simulink model "TwoScaleSimulation"  (R2021b)
settings: Solver=ode15s  StartTime=0.0  StopTime=1440*2  RelTol=1e-5
model workspace (MAT data in the model file):
  K_ACTH_StARp37 = 21.62
  k21 = 3080
  k_ACORT = 44.5
  k_StARp37 = 0.778
  ke = 0.099
  mu_StARp37 = 19.8
settings Model: Creator=Mahdi  LastModifiedBy=Mahdi
settings SolverCC: AlgebraicLoopSolver=TrustRegion
settings DebuggingCC: SFMachineParentedDataDiag=warning

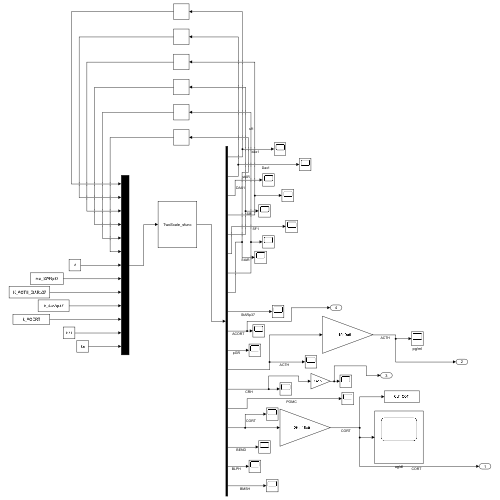
[thumbnail: Simulink's stored preview of the top-level diagram]
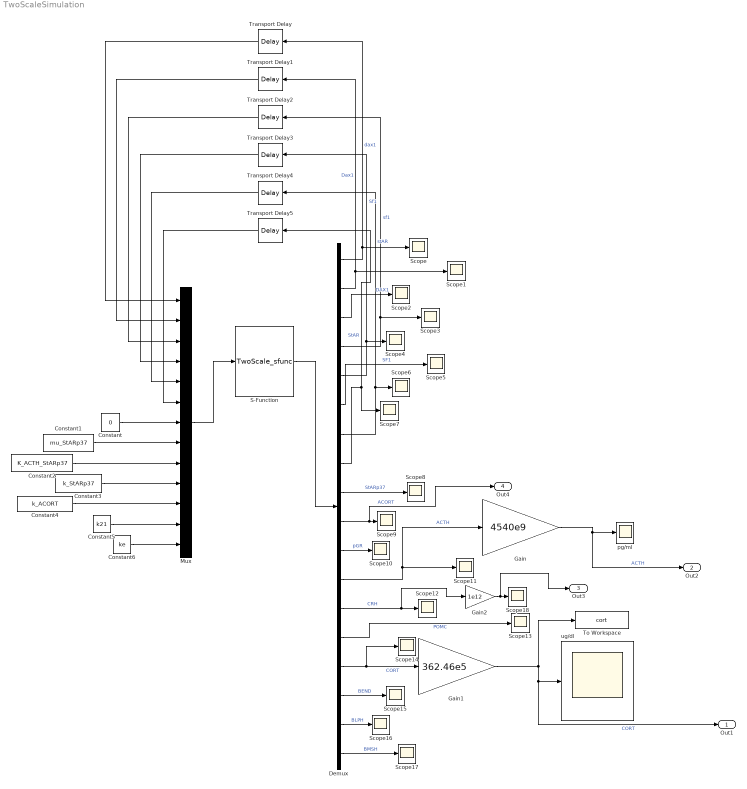
== system TwoScaleSimulation ==
  Constant : Constant  Value=0
  Constant1 : Constant  Value=mu_StARp37
  Constant2 : Constant  Value=K_ACTH_StARp37
  Constant3 : Constant  Value=k_StARp37
  Constant4 : Constant  Value=k_ACORT
  Constant5 : Constant  Value=k21
  Constant6 : Constant  Value=ke
  Demux : Demux  Outputs=18
  Gain : Gain  Gain=4540e9
  Gain1 : Gain  Gain=362.46e5
  Gain2 : Gain  Gain=1e12
  Mux : Mux  Inputs=13
  S-Function : S-Function  FunctionName=TwoScale_sfunc  SFunctionDeploymentMode=off  EnableBusSupport=off
  Scope{,1..18} (19 alike) : Scope
  To Workspace : ToWorkspace  VariableName=cort  SampleTime=10
  Transport Delay : TransportDelay  DelayTime=2.79
  Transport Delay1 : TransportDelay  DelayTime=1.4
  Transport Delay2 : TransportDelay  DelayTime=14.75
  Transport Delay3 : TransportDelay  DelayTime=1.38
  Transport Delay4 : TransportDelay  DelayTime=5.58
  Transport Delay5 : TransportDelay
  pg/ml : Scope
  ug/dl : Scope
  Out1 : Outport
  Out2 : Outport  Port=2
  Out3 : Outport  Port=3
  Out4 : Outport  Port=4
  wires:
  Demux/10 -> Out4/1, Scope9/1  "ACORT"
  Demux/6 -> Scope5/1  "SF1"
  Demux/7 -> Transport Delay4/1, Scope6/1  "stAR"
  Demux/2 -> Transport Delay1/1, Scope1/1  "Dax1"
  Demux/4 -> Transport Delay2/1, Scope3/1  "sf1"
  Mux/1 -> S-Function/1
  Transport Delay4/1 -> Mux/5
  Transport Delay1/1 -> Mux/2
  Transport Delay/1 -> Mux/1
  Demux/11 -> Scope10/1  "pGR"
  Transport Delay5/1 -> Mux/6
  Demux/8 -> Scope7/1, Transport Delay5/1  "StAR"
  Demux/9 -> Scope8/1  "StARp37"
  S-Function/1 -> Demux/1
  Transport Delay3/1 -> Mux/4
  Demux/3 -> Scope2/1  "DAX1"
  Demux/1 -> Transport Delay/1, Scope/1  "dax1"
  Demux/5 -> Transport Delay3/1, Scope4/1  "Sf1"
  Transport Delay2/1 -> Mux/3
  Demux/12 -> Scope11/1, Gain/1  "ACTH"
  Demux/13 -> Gain2/1, Scope12/1  "CRH"
  Demux/14 -> Scope13/1  "POMC"
  Demux/15 -> Scope14/1, Gain1/1  "CORT"
  Gain/1 -> Out2/1, pg/ml/1  "ACTH"
  Gain1/1 -> ug/dl/1, Out1/1, To Workspace/1  "CORT"
  Constant/1 -> Mux/7
  Demux/16 -> Scope15/1  "BEND"
  Demux/17 -> Scope16/1  "BLPH"
  Demux/18 -> Scope17/1  "BMSH"
  Constant1/1 -> Mux/8
  Constant2/1 -> Mux/9
  Constant3/1 -> Mux/10
  Constant4/1 -> Mux/11
  Constant5/1 -> Mux/12
  Constant6/1 -> Mux/13
  Gain2/1 -> Out3/1, Scope18/1
